simulink model "newStuff"  (R2015a)
settings: Solver=ode8  SolverMode=SingleTasking  StartTime=0  StopTime=25  FixedStep=.05  RelTol=1e-3
InitFcn:
  | fclose(instrfind);
  | s = serial('COM4');
  | set(s, 'DataBits', 8);
  | set(s, 'StopBits', 1);
  | set(s, 'BaudRate', 230400);
  | set(s, 'Parity', 'none');
  | fopen(s);
  | a='b';
  | while a~='a'
  |     a=fread(s,1,'uchar');
  | end
  | fprintf(s,'%c','a');
  | fscanf(s,'%u');
StopFcn:
  | fprintf(s,'1,0,0');
  | flushinput(s);
undefined symbols (not defined in the file or in its folder): fgetl, sscanf
libraries: simulink x1, sldrtlib x1
settings Model: ExtModeTrigDuration=2  Creator=ICPUB401  LastModifiedBy=zammi
settings SolverCC: InsertRTBMode=Always
settings DataIOCC: SaveOutput=off
settings OptimizationCC: OptimizeModelRefInitCode=on  LifeSpan=1
settings DebuggingCC: UnderspecifiedInitializationDetection=Classic  MergeDetectMultiDrivingBlocksExec=none  InheritedTsInSrcMsg=none
settings HardwareCC: ProdBitPerInt=16  ProdBitPerPointer=8  ProdIntDivRoundTo=Zero  ProdEndianess=LittleEndian  ProdWordSize=8  ProdHWDeviceType=Atmel->AVR
settings RTWCC: SystemTargetFile=realtime.tlc  GenerateMakefile=off  TemplateMakefile=realtime.tmf  Description=Run on Target Hardware  RTWVerbose=off
settings ERTTargetCC: CombineOutputUpdateFcns=off  ExtModeTransport=3  ExtModeMexFile=ext_serial_win32_comm_rtt  ExtModeMexArgs=0 1 9600  ERTSrcFileBannerTemplate=realtime_code_template.cgt  ERTHdrFileBannerTemplate=realtime_code_template.cgt  ERTDataSrcFileTemplate=realtime_code_template.cgt  ERTDataHdrFileTemplate=realtime_code_template.cgt  ERTCustomFileTemplate=realtime_file_process.tlc

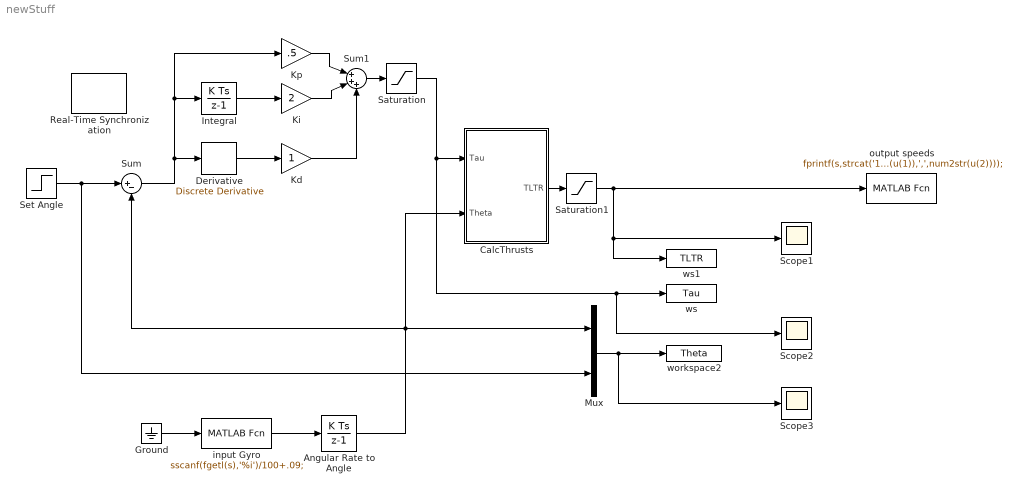
== system newStuff ==
  Angular Rate to Angle : DiscreteIntegrator  InitialConditionSetting=State (most efficient)  SampleTime=.05
  CalcThrusts : MATLAB Function  TreatAsAtomicUnit=on
  Derivative : simulink/Discrete/Discrete Derivative  gainval=1.0  ICPrevScaledInput=0.0  InputProcessing=Inherited  OutMin=[]  OutMax=[]  OutDataType=fixdt(1, 16)  OutScaling=2^-10  DoSatur=off
  Ground : Ground
  Integral : DiscreteIntegrator  InitialConditionSetting=State (most efficient)  SampleTime=.05
  Kd : Gain
  Ki : Gain  Gain=2
  Kp : Gain  Gain=.5
  Mux : Mux  Inputs=2
  Real-Time Synchronization : sldrtlib/Real-Time Synchronization  SampleTime=-1  MaxMissedTicks=10  ShowMissedTicks=off  YieldWhenWaiting=on
  Saturation : Saturate  UpperLimit=.75  LowerLimit=-.75
  Saturation1 : Saturate  UpperLimit=180  LowerLimit=0
  Scope1 : Scope
      settings: YMin=0  YMax=180
  Scope2 : Scope
      settings: YMin=-1  YMax=1  SaveName=ScopeData2
  Scope3 : Scope
      settings: YMin=-1.570796326794897  YMax=1.570796326794897
  Set Angle : Step  Time=5  After=10*pi/180
  Sum : Sum  Inputs=|+-
  Sum1 : Sum  Inputs=|+++
  input Gyro : MATLABFcn  Priority=1  MATLABFcn=sscanf(fgetl(s),'%i')/100+.09;  OutputDimensions=1  OutputSignalType=real
      settings: CloseFcn=flushinput(s);
  output speeds : MATLABFcn  MATLABFcn=fprintf(s,strcat('1,',num2str(u(1)),',',num2str(u(2))));  OutputDimensions=0  OutputSignalType=real
  workspace2 : ToWorkspace  VariableName=Theta  SampleTime=-1
      settings: Save2DSignal=2-D array (concatenate along first dimension)
  ws : ToWorkspace  VariableName=Tau  SampleTime=-1
      settings: Save2DSignal=2-D array (concatenate along first dimension)
  "ws1 " : ToWorkspace  VariableName=TLTR  SampleTime=-1
      settings: Save2DSignal=2-D array (concatenate along first dimension)
  wires:
  Sum1/1 -> Saturation/1
  Saturation1/1 -> Scope1/1, "ws1 "/1, output speeds/1
  Derivative/1 -> Kd/1
  Integral/1 -> Ki/1
  Ground/1 -> input Gyro/1
  input Gyro/1 -> Angular Rate to Angle/1
  Ki/1 -> Sum1/2
  Kd/1 -> Sum1/3
  Kp/1 -> Sum1/1
  Angular Rate to Angle/1 -> Mux/1, CalcThrusts/2(Theta), Sum/2
  CalcThrusts/1(TLTR) -> Saturation1/1
  Set Angle/1 -> Sum/1, Mux/2
  Sum/1 -> Derivative/1, Integral/1, Kp/1
  Saturation/1 -> ws/1, Scope2/1, CalcThrusts/1(Tau)
  Mux/1 -> Scope3/1, workspace2/1

== matlab function newStuff/CalcThrusts ==
  data: Tau input; TLTR output; Theta input
function TLTR  = fcn(Tau,Theta)
%#codegen
weight = .2*9.81;
l = .45;
TLTR = zeros(2,1);
T = [cos(Theta), cos(Theta); -l/2, l/2]\[weight;Tau];
TLTR(1) = round(60*T(1)/(.520*9.81))+80;
TLTR(2) = round(60*T(2)/(.520*9.81))+80;
